simulink model "SWC_AFE_Control"  (R2022b)
settings: configuration reference "DC_DC_Charger_Configuration" (kept outside this file)
undefined symbols (not defined in the file or in its folder): DUTY_COUNT_LOWER_LMIT, DUTY_COUNT_UPPER_LMIT, Fault_Counts_perms, GRID_NORM_FREQ, GRID_VOLT_ADC_OFFSET, HALF_DUTY_PERIOD, INDUCTANCE, PI, PLL_FREQ_LOW_LIMIT, PLL_FREQ_UPP_LIMIT, PLL_PI_INTGRL_RESET, PLL_PI_KI, PLL_PI_KP, PLL_PI_LOWER_LIMIT, PLL_PI_UPPER_LIMIT, PLL_RATE, PLL_VD_ERROR_LIMIT, PLL_VD_ESTIMETED, PLL_VQ_ERROR_LIMIT, VDC_LOWER_LIM_SVPWM, VDC_UPPER_LIM_SVPWM
libraries: simulink x13, common_lib x8
(part 2 of 2)

== system SWC_AFE_Control/PWM_Loop/PLL/PLL_Lock_Detection_Block ==
  d_actual : Inport
  Vq_error : Inport  Port=2
  Abs : Abs  SaturateOnIntegerOverflow=off
  Abs1 : Abs  SaturateOnIntegerOverflow=off
  Add3 : Sum  Inputs=+-
  Constant1 : Constant  Value=PLL_VD_ESTIMETED  OutDataTypeStr=single  SampleTime=-1
  Constant12 : Constant  Value=PLL_VD_ERROR_LIMIT  OutDataTypeStr=single  SampleTime=-1
  Constant9 : Constant  Value=PLL_VQ_ERROR_LIMIT  OutDataTypeStr=single  SampleTime=-1
  Data Type Conversion : DataTypeConversion  OutDataTypeStr=single  SaturateOnIntegerOverflow=off  RndMeth=Floor
  Debounce1 : Subsystem  mask{Fault_Time_ms=40}
      mask DialogControl ParameterGroupVar Prompt: Fault Debounce time (msec)
  Logical Operator : Logic  AllPortsSameDT=off  OutDataTypeStr=boolean
  Relational Operator : RelationalOperator  Operator=<=  OutDataTypeStr=boolean  RndMeth=Simplest  InputSameDT=off
  Relational Operator2 : RelationalOperator  Operator=<=  OutDataTypeStr=boolean  RndMeth=Simplest  InputSameDT=off
  Switch2 : Switch  Threshold=0.5  SaturateOnIntegerOverflow=off  InputSameDT=off
  PLL_lock_out : Outport
  wires:
  Debounce1/1(Fault_Out) -> Switch2/1
  Switch2/1 -> PLL_lock_out/1
  Abs1/1 -> Relational Operator2/1
  Add3/1 -> Abs1/1
  Constant1/1 -> Add3/2
  d_actual/1 -> Add3/1
  Abs/1 -> Relational Operator/1
  Relational Operator/1 -> Logical Operator/2
  Relational Operator2/1 -> Logical Operator/1
  Constant12/1 -> Relational Operator2/2
  Constant9/1 -> Relational Operator/2
  Logical Operator/1 -> Data Type Conversion/1
  Vq_error/1 -> Abs/1
  Data Type Conversion/1 -> Debounce1/1(Fault_In), Switch2/2, Switch2/3

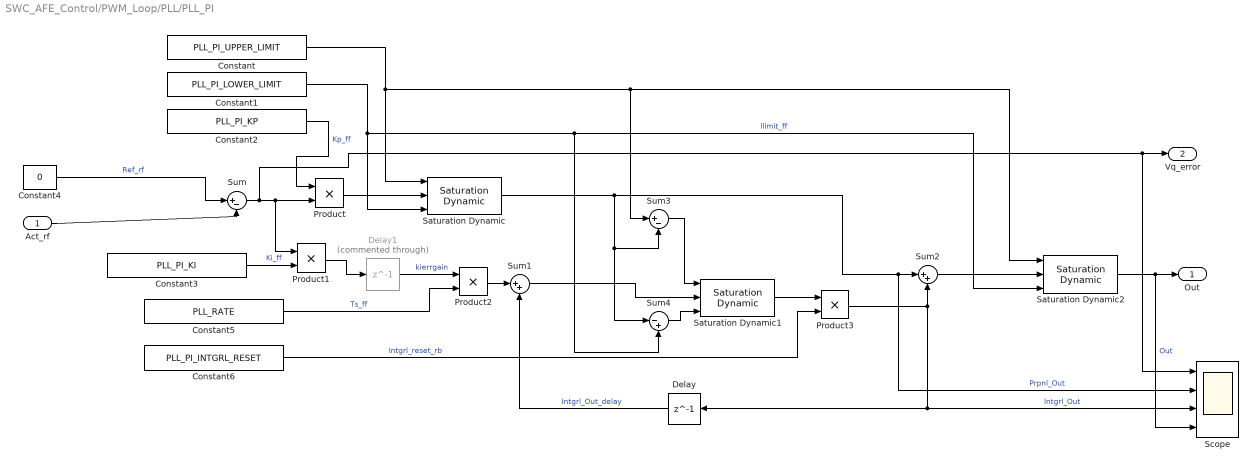
== system SWC_AFE_Control/PWM_Loop/PLL/PLL_PI ==
  Act_rf : Inport
  Constant : Constant  Value=PLL_PI_UPPER_LIMIT  SampleTime=-1
  Constant1 : Constant  Value=PLL_PI_LOWER_LIMIT  SampleTime=-1
  Constant2 : Constant  Value=PLL_PI_KP  SampleTime=-1
  Constant3 : Constant  Value=PLL_PI_KI  SampleTime=-1
  Constant4 : Constant  Value=0  SampleTime=-1
  Constant5 : Constant  Value=PLL_RATE  SampleTime=-1
  Constant6 : Constant  Value=PLL_PI_INTGRL_RESET  SampleTime=-1
  Delay : Delay  DelayLength=1
  Delay1 : Delay  Commented=through  DelayLength=1
  Product{,1..3} (4 alike) : Product
  Saturation Dynamic : simulink/Discontinuities/Saturation Dynamic  OutMin=[]  OutMax=[]  OutDataTypeStr=Inherit: Same as second input  OutDataType=fixdt(1, 16)  OutScaling=2^-10  DoSatur=off
  Saturation Dynamic1 : simulink/Discontinuities/Saturation Dynamic  OutMin=[]  OutMax=[]  OutDataTypeStr=Inherit: Same as second input  OutDataType=fixdt(1, 16)  OutScaling=2^-10  DoSatur=off
  Saturation Dynamic2 : simulink/Discontinuities/Saturation Dynamic  OutMin=[]  OutMax=[]  OutDataTypeStr=Inherit: Same as second input  OutDataType=fixdt(1, 16)  OutScaling=2^-10  DoSatur=off
  Scope : Scope  NumInputPorts=4
  Sum : Sum  Inputs=|+-
  Sum1 : Sum  Inputs=|++
  Sum2 : Sum  Inputs=|++
  Sum3 : Sum  Inputs=|+-
  Sum4 : Sum  Inputs=|-+
  Out : Outport
  Vq_error : Outport  Port=2
  wires:
  Sum/1 -> Scope/1, Vq_error/1, Product/2, Product1/1
  Constant5/1 -> Product2/2  "Ts_ff"
  Constant6/1 -> Product3/2  "Intgrl_reset_rb"
  Sum1/1 -> Saturation Dynamic1/2
  Product2/1 -> Sum1/1
  Product1/1 -> Delay1/1
  Saturation Dynamic2/1 -> Scope/4, Out/1  "Out"
  Delay1/1 -> Product2/1  "kierrgain"
  Saturation Dynamic1/1 -> Product3/1
  Sum3/1 -> Saturation Dynamic1/1
  Constant4/1 -> Sum/1  "Ref_rf"
  Sum4/1 -> Saturation Dynamic1/3
  Saturation Dynamic/1 -> Scope/2, Sum2/1, Sum3/2, Sum4/1  "Prpnl_Out"
  Delay/1 -> Sum1/2  "Intgrl_Out_delay"
  Sum2/1 -> Saturation Dynamic2/2
  Product/1 -> Saturation Dynamic/2
  Constant2/1 -> Product/1  "Kp_ff"
  Act_rf/1 -> Sum/2
  Product3/1 -> Scope/3, Delay/1, Sum2/2  "Intgrl_Out"
  Constant/1 -> Saturation Dynamic2/1, Sum3/1, Saturation Dynamic/1
  Constant3/1 -> Product1/2  "Ki_ff"
  Constant1/1 -> Sum4/2, Saturation Dynamic2/3, Saturation Dynamic/3  "llimit_ff"

== system SWC_AFE_Control/PWM_Loop/PLL/SOGI ==
  vg : Inport
  omega : Inport  Port=2
  Add : Sum  Inputs=+-  OutDataTypeStr=single
  Add1 : Sum
  Add2 : Sum  OutDataTypeStr=single
  Add3 : Sum  Inputs=-+  OutDataTypeStr=single
  Constant : Constant  Value=PLL_RATE  OutDataTypeStr=single  SampleTime=-1
  Delay{,1..3} (4 alike) : Delay  DelayLength=1
  Gain : Gain
  Product : Product
  Product1 : Product
  Product2 : Product
  vg_al : Outport
  vg_be : Outport  Port=2
  wires:
  omega/1 -> Product2/1  "omega"
  Product2/1 -> Product1/1, Product/2
  Constant/1 -> Product2/2
  Delay3/1 -> Add3/1
  Add3/1 -> Gain/1
  vg/1 -> Add3/2  "vg"
  Gain/1 -> Add/1
  Delay2/1 -> Add/2
  Delay1/1 -> Add2/1
  Product1/1 -> Add2/2
  Delay/1 -> Add1/2
  Product/1 -> Add1/1
  Add/1 -> Product/1
  Add1/1 -> vg_al/1, Delay3/1, Delay/1, Product1/2  "vg_al"
  Add2/1 -> vg_be/1, Delay1/1, Delay2/1  "vg_be"

== system SWC_AFE_Control/PWM_Loop/PLL/SOGI1 ==
  vg : Inport
  omega : Inport  Port=2
  Add : Sum  Inputs=+-  OutDataTypeStr=single
  Add1 : Sum
  Add2 : Sum  OutDataTypeStr=single
  Add3 : Sum  Inputs=-+  OutDataTypeStr=single
  Constant : Constant  Value=PLL_RATE  OutDataTypeStr=single  SampleTime=-1
  Delay{,1..3} (4 alike) : Delay  DelayLength=1
  Gain : Gain
  Product : Product
  Product1 : Product
  Product2 : Product
  vg_al : Outport
  vg_be : Outport  Port=2
  wires:
  Delay/1 -> Add1/2
  Delay3/1 -> Add3/1
  Gain/1 -> Add/1
  vg/1 -> Add3/2  "vg"
  Constant/1 -> Product2/2
  Add2/1 -> vg_be/1, Delay1/1, Delay2/1  "vg_be"
  Add3/1 -> Gain/1
  Product2/1 -> Product1/1, Product/2
  omega/1 -> Product2/1  "omega"
  Product1/1 -> Add2/2
  Product/1 -> Add1/1
  Delay2/1 -> Add/2
  Delay1/1 -> Add2/1
  Add/1 -> Product/1
  Add1/1 -> vg_al/1, Delay3/1, Delay/1, Product1/2  "vg_al"

== system SWC_AFE_Control/PWM_Loop/PLL/abctoalphabeta ==
  ph_a : Inport
  ph_b : Inport  Port=2
  ph_c : Inport  Port=3
  Gain1 : Gain  Gain=1/2
  Gain2 : Gain
  Gain3 : Gain  Gain=1/2
  Gain4 : Gain  Gain=sqrt(3)/2
  Sum : Sum  Inputs=|+--
  Sum5 : Sum  Inputs=|+-
  alpha : Outport
  beta : Outport  Port=2
  wires:
  Gain4/1 -> beta/1
  ph_a/1 -> Sum/1
  Gain3/1 -> Sum/3
  Gain2/1 -> alpha/1
  ph_c/1 -> Gain3/1, Sum5/2
  ph_b/1 -> Gain1/1, Sum5/1
  Sum5/1 -> Gain4/1
  Gain1/1 -> Sum/2
  Sum/1 -> Gain2/1

== system SWC_AFE_Control/PWM_Loop/PLL/alphabetatodq ==
  alpha : Inport
  beta : Inport  Port=2
  sinthetha : Inport  Port=3
  costhetha : Inport  Port=4
  Product{1..4} (4 alike) : Product
  Sum : Sum  Inputs=|++
  Sum5 : Sum  Inputs=|-+
  d : Outport
  q : Outport  Port=2
  wires:
  Product4/1 -> Sum5/2
  Product2/1 -> Sum5/1
  Product1/1 -> Sum/2
  Product3/1 -> Sum/1
  sinthetha/1 -> Product1/1, Product2/2
  beta/1 -> Product1/2, Product4/2
  costhetha/1 -> Product3/2, Product4/1
  alpha/1 -> Product3/1, Product2/1
  Sum5/1 -> q/1
  Sum/1 -> d/1

== system SWC_AFE_Control/PWM_Loop/PWM_DUTY/Subsystem ==
  In1 : Inport
  Add5 : Sum
  Constant7 : Constant  Value=HALF_DUTY_PERIOD
  Data Type Conversion : DataTypeConversion  OutDataTypeStr=single  SaturateOnIntegerOverflow=off  RndMeth=Floor
  Gain5 : Gain  Gain=HALF_DUTY_PERIOD
  Out1 : Outport
  wires:
  In1/1 -> Gain5/1
  Gain5/1 -> Add5/1
  Constant7/1 -> Add5/2
  Add5/1 -> Data Type Conversion/1
  Data Type Conversion/1 -> Out1/1

== system SWC_AFE_Control/PWM_Loop/PWM_DUTY/Subsystem1 ==
  In1 : Inport
  Add5 : Sum
  Constant7 : Constant  Value=HALF_DUTY_PERIOD
  Data Type Conversion : DataTypeConversion  OutDataTypeStr=single  SaturateOnIntegerOverflow=off  RndMeth=Floor
  Gain5 : Gain  Gain=HALF_DUTY_PERIOD
  Out1 : Outport
  wires:
  In1/1 -> Gain5/1
  Gain5/1 -> Add5/1
  Constant7/1 -> Add5/2
  Add5/1 -> Data Type Conversion/1
  Data Type Conversion/1 -> Out1/1

== system SWC_AFE_Control/PWM_Loop/PWM_DUTY/Subsystem2 ==
  In1 : Inport
  Add5 : Sum
  Constant7 : Constant  Value=HALF_DUTY_PERIOD
  Data Type Conversion : DataTypeConversion  OutDataTypeStr=single  SaturateOnIntegerOverflow=off  RndMeth=Floor
  Gain5 : Gain  Gain=HALF_DUTY_PERIOD
  Out1 : Outport
  wires:
  In1/1 -> Gain5/1
  Gain5/1 -> Add5/1
  Constant7/1 -> Add5/2
  Add5/1 -> Data Type Conversion/1
  Data Type Conversion/1 -> Out1/1

== system SWC_AFE_Control/Control_Loop/CONTROL/abctodq/abctoalphabeta ==
  ph_a : Inport
  ph_b : Inport  Port=2
  ph_c : Inport  Port=3
  Gain1 : Gain  Gain=1/2
  Gain2 : Gain  Gain=2/3
  Gain3 : Gain  Gain=1/2
  Gain4 : Gain  Gain=sqrt(3)/2*2/3
  Sum : Sum  Inputs=|+--
  Sum5 : Sum  Inputs=|+-
  alpha : Outport
  beta : Outport  Port=2
  wires:
  Sum/1 -> Gain2/1
  Gain1/1 -> Sum/2
  Sum5/1 -> Gain4/1
  ph_b/1 -> Sum5/1, Gain1/1
  ph_c/1 -> Sum5/2, Gain3/1
  Gain2/1 -> alpha/1
  Gain3/1 -> Sum/3
  ph_a/1 -> Sum/1
  Gain4/1 -> beta/1

== system SWC_AFE_Control/Control_Loop/CONTROL/abctodq/alphabetatodq ==
  alpha : Inport
  beta : Inport  Port=2
  sinthetha : Inport  Port=3
  costhetha : Inport  Port=4
  Product{1..4} (4 alike) : Product
  Sum : Sum  Inputs=|++
  Sum5 : Sum  Inputs=|-+
  d : Outport
  q : Outport  Port=2
  wires:
  Sum/1 -> d/1
  Sum5/1 -> q/1
  alpha/1 -> Product2/1, Product3/1
  costhetha/1 -> Product4/1, Product3/2
  beta/1 -> Product4/2, Product1/2
  sinthetha/1 -> Product2/2, Product1/1
  Product3/1 -> Sum/1
  Product1/1 -> Sum/2
  Product2/1 -> Sum5/1
  Product4/1 -> Sum5/2

== system SWC_AFE_Control/Control_Loop/CONTROL/dqtoabc/alphabetatoabc ==
  Input : Inport
  Input1 : Inport  Port=2
  Gain1 : Gain  Gain=sqrt(3)/2
  Gain3 : Gain  Gain=1/2
  Sum : Sum  Inputs=|+-  AccumDataTypeStr=single  OutDataTypeStr=single
  Sum5 : Sum  Inputs=|--  AccumDataTypeStr=single  OutDataTypeStr=single
  ph_a : Outport
  ph_b : Outport  Port=2
  ph_c : Outport  Port=3
  wires:
  Sum5/1 -> ph_c/1
  Input1/1 -> Gain1/1
  Input/1 -> Gain3/1, ph_a/1
  Sum/1 -> ph_b/1
  Gain1/1 -> Sum5/1, Sum/1
  Gain3/1 -> Sum/2, Sum5/2

== system SWC_AFE_Control/Control_Loop/CONTROL/dqtoabc/dqtoalphabeta ==
  Input2 : Inport
  Input3 : Inport  Port=2
  Input1 : Inport  Port=3
  Input : Inport  Port=4
  Product{1..4} (4 alike) : Product
  Sum : Sum  Inputs=|+-  AccumDataTypeStr=single  OutDataTypeStr=single
  Sum5 : Sum  Inputs=|++  AccumDataTypeStr=single  OutDataTypeStr=single
  alpha : Outport
  beta : Outport  Port=2
  wires:
  Sum/1 -> alpha/1
  Sum5/1 -> beta/1
  Input2/1 -> Product2/1, Product3/1
  Input/1 -> Product4/1, Product3/2
  Input3/1 -> Product4/2, Product1/2
  Input1/1 -> Product2/2, Product1/1
  Product3/1 -> Sum/1
  Product1/1 -> Sum/2
  Product2/1 -> Sum5/1
  Product4/1 -> Sum5/2

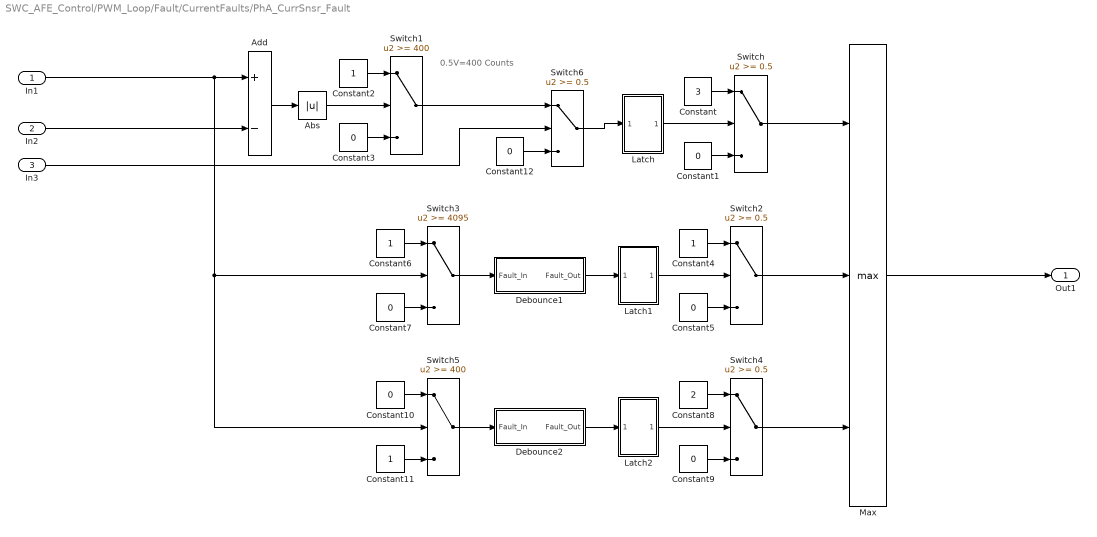
== system SWC_AFE_Control/PWM_Loop/Fault/CurrentFaults/PhA_CurrSnsr_Fault ==
  note: 0.5V=400 Counts
  In1 : Inport
  In2 : Inport  Port=2
  In3 : Inport  Port=3
  Abs : Abs  SaturateOnIntegerOverflow=off
  Add : Sum  Inputs=+-
  Constant : Constant  Value=3
  Constant{1,3,5,7,9..10,12} (7 alike) : Constant  Value=0
  Constant{2,4,6,11} (4 alike) : Constant
  Constant8 : Constant  Value=2
  Debounce1 : Subsystem  mask{Fault_Time_ms=4}
      mask DialogControl ParameterGroupVar Prompt: Fault Debounce time (msec)
  Debounce2 : Subsystem  mask{Fault_Time_ms=4}
      mask DialogControl ParameterGroupVar Prompt: Fault Debounce time (msec)
  Latch : Subsystem
  Latch1 : Subsystem
  Latch2 : Subsystem
  Max : MinMax  Function=max  Inputs=3
  Switch{,2,4,6} (4 alike) : Switch  Threshold=0.5  SaturateOnIntegerOverflow=off  InputSameDT=off
  Switch1 : Switch  Threshold=400  SaturateOnIntegerOverflow=off  InputSameDT=off
  Switch3 : Switch  Threshold=4095  SaturateOnIntegerOverflow=off  InputSameDT=off
  Switch5 : Switch  Threshold=400  SaturateOnIntegerOverflow=off  InputSameDT=off
  Out1 : Outport
  wires:
  Constant6/1 -> Switch3/1
  Switch1/1 -> Switch6/1
  Constant2/1 -> Switch1/1
  Switch/1 -> Max/1
  Constant7/1 -> Switch3/3
  Debounce1/1(Fault_Out) -> Latch1/1(In1)
  Switch3/1 -> Debounce1/1(Fault_In)
  Constant4/1 -> Switch2/1
  Latch1/1(Out1) -> Switch2/2
  Constant5/1 -> Switch2/3
  Switch6/1 -> Latch/1(In1)
  Add/1 -> Abs/1
  Constant/1 -> Switch/1
  Constant1/1 -> Switch/3
  Constant8/1 -> Switch4/1
  Constant11/1 -> Switch5/3
  Latch/1(Out1) -> Switch/2
  Constant9/1 -> Switch4/3
  Latch2/1(Out1) -> Switch4/2
  Debounce2/1(Fault_Out) -> Latch2/1(In1)
  In1/1 -> Switch5/2, Switch3/2, Add/1
  Switch4/1 -> Max/3
  Switch2/1 -> Max/2
  Constant3/1 -> Switch1/3
  Constant12/1 -> Switch6/3
  Switch5/1 -> Debounce2/1(Fault_In)
  Constant10/1 -> Switch5/1
  Abs/1 -> Switch1/2
  In2/1 -> Add/2
  Max/1 -> Out1/1
  In3/1 -> Switch6/2

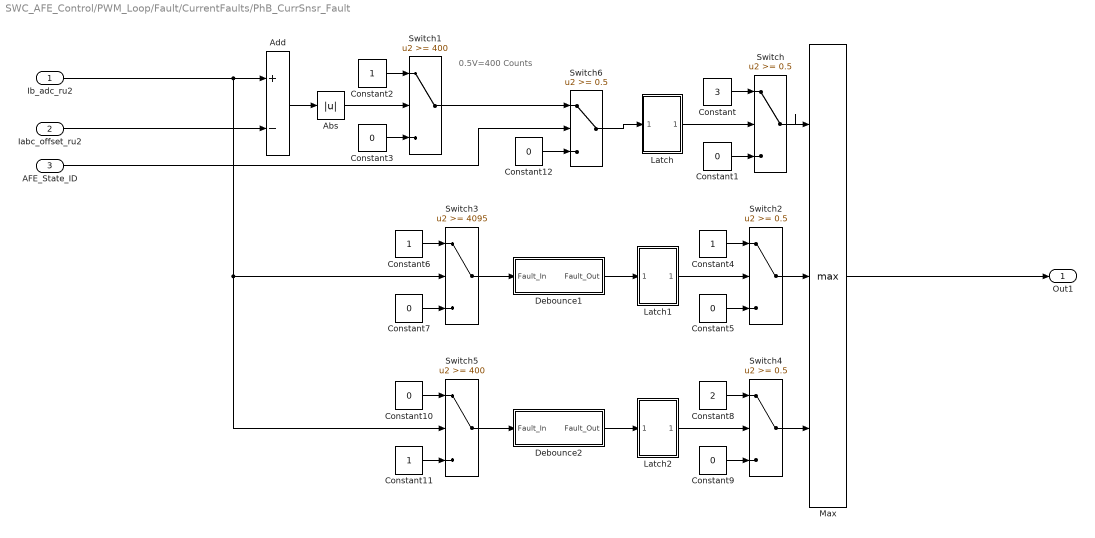
== system SWC_AFE_Control/PWM_Loop/Fault/CurrentFaults/PhB_CurrSnsr_Fault ==
  note: 0.5V=400 Counts
  Ib_adc_ru2 : Inport
  Iabc_offset_ru2 : Inport  Port=2
  AFE_State_ID : Inport  Port=3
  Abs : Abs  SaturateOnIntegerOverflow=off
  Add : Sum  Inputs=+-
  Constant : Constant  Value=3
  Constant{1,3,5,7,9..10,12} (7 alike) : Constant  Value=0
  Constant{2,4,6,11} (4 alike) : Constant
  Constant8 : Constant  Value=2
  Debounce1 : Subsystem  mask{Fault_Time_ms=4}
      mask DialogControl ParameterGroupVar Prompt: Fault Debounce time (msec)
  Debounce2 : Subsystem  mask{Fault_Time_ms=4}
      mask DialogControl ParameterGroupVar Prompt: Fault Debounce time (msec)
  Latch : Subsystem
  Latch1 : Subsystem
  Latch2 : Subsystem
  Max : MinMax  Function=max  Inputs=3
  Switch{,2,4,6} (4 alike) : Switch  Threshold=0.5  SaturateOnIntegerOverflow=off  InputSameDT=off
  Switch1 : Switch  Threshold=400  SaturateOnIntegerOverflow=off  InputSameDT=off
  Switch3 : Switch  Threshold=4095  SaturateOnIntegerOverflow=off  InputSameDT=off
  Switch5 : Switch  Threshold=400  SaturateOnIntegerOverflow=off  InputSameDT=off
  Out1 : Outport
  wires:
  Constant6/1 -> Switch3/1
  Switch1/1 -> Switch6/1
  Constant2/1 -> Switch1/1
  Switch/1 -> Max/1
  Constant7/1 -> Switch3/3
  Debounce1/1(Fault_Out) -> Latch1/1(In1)
  Switch3/1 -> Debounce1/1(Fault_In)
  Constant4/1 -> Switch2/1
  Latch1/1(Out1) -> Switch2/2
  Constant5/1 -> Switch2/3
  Switch6/1 -> Latch/1(In1)
  Add/1 -> Abs/1
  Constant/1 -> Switch/1
  Constant1/1 -> Switch/3
  Constant8/1 -> Switch4/1
  Constant11/1 -> Switch5/3
  Latch/1(Out1) -> Switch/2
  Constant9/1 -> Switch4/3
  Latch2/1(Out1) -> Switch4/2
  Debounce2/1(Fault_Out) -> Latch2/1(In1)
  Ib_adc_ru2/1 -> Switch5/2, Switch3/2, Add/1
  Switch4/1 -> Max/3
  Switch2/1 -> Max/2
  Constant3/1 -> Switch1/3
  Constant12/1 -> Switch6/3
  Switch5/1 -> Debounce2/1(Fault_In)
  Constant10/1 -> Switch5/1
  Abs/1 -> Switch1/2
  Iabc_offset_ru2/1 -> Add/2
  Max/1 -> Out1/1
  AFE_State_ID/1 -> Switch6/2

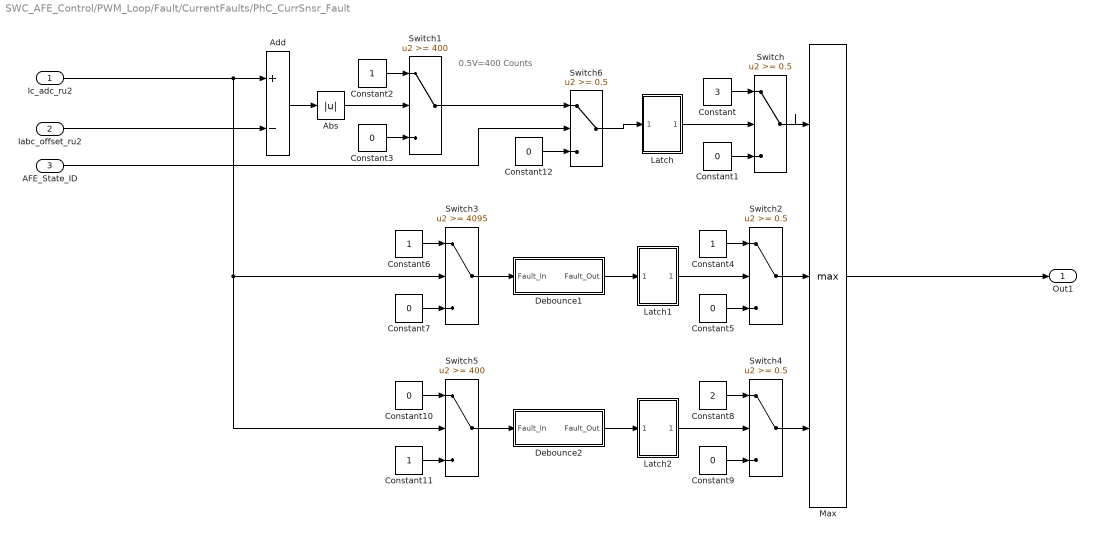
== system SWC_AFE_Control/PWM_Loop/Fault/CurrentFaults/PhC_CurrSnsr_Fault ==
  note: 0.5V=400 Counts
  Ic_adc_ru2 : Inport
  Iabc_offset_ru2 : Inport  Port=2
  AFE_State_ID : Inport  Port=3
  Abs : Abs  SaturateOnIntegerOverflow=off
  Add : Sum  Inputs=+-
  Constant : Constant  Value=3
  Constant{1,3,5,7,9..10,12} (7 alike) : Constant  Value=0
  Constant{2,4,6,11} (4 alike) : Constant
  Constant8 : Constant  Value=2
  Debounce1 : Subsystem  mask{Fault_Time_ms=4}
      mask DialogControl ParameterGroupVar Prompt: Fault Debounce time (msec)
  Debounce2 : Subsystem  mask{Fault_Time_ms=4}
      mask DialogControl ParameterGroupVar Prompt: Fault Debounce time (msec)
  Latch : Subsystem
  Latch1 : Subsystem
  Latch2 : Subsystem
  Max : MinMax  Function=max  Inputs=3
  Switch{,2,4,6} (4 alike) : Switch  Threshold=0.5  SaturateOnIntegerOverflow=off  InputSameDT=off
  Switch1 : Switch  Threshold=400  SaturateOnIntegerOverflow=off  InputSameDT=off
  Switch3 : Switch  Threshold=4095  SaturateOnIntegerOverflow=off  InputSameDT=off
  Switch5 : Switch  Threshold=400  SaturateOnIntegerOverflow=off  InputSameDT=off
  Out1 : Outport
  wires:
  Constant6/1 -> Switch3/1
  Switch1/1 -> Switch6/1
  Constant2/1 -> Switch1/1
  Switch/1 -> Max/1
  Constant7/1 -> Switch3/3
  Debounce1/1(Fault_Out) -> Latch1/1(In1)
  Switch3/1 -> Debounce1/1(Fault_In)
  Constant4/1 -> Switch2/1
  Latch1/1(Out1) -> Switch2/2
  Constant5/1 -> Switch2/3
  Switch6/1 -> Latch/1(In1)
  Add/1 -> Abs/1
  Constant/1 -> Switch/1
  Constant1/1 -> Switch/3
  Constant8/1 -> Switch4/1
  Constant11/1 -> Switch5/3
  Latch/1(Out1) -> Switch/2
  Constant9/1 -> Switch4/3
  Latch2/1(Out1) -> Switch4/2
  Debounce2/1(Fault_Out) -> Latch2/1(In1)
  Ic_adc_ru2/1 -> Switch5/2, Switch3/2, Add/1
  Switch4/1 -> Max/3
  Switch2/1 -> Max/2
  Constant3/1 -> Switch1/3
  Constant12/1 -> Switch6/3
  Switch5/1 -> Debounce2/1(Fault_In)
  Constant10/1 -> Switch5/1
  Abs/1 -> Switch1/2
  Iabc_offset_ru2/1 -> Add/2
  Max/1 -> Out1/1
  AFE_State_ID/1 -> Switch6/2

== system SWC_AFE_Control/PWM_Loop/PLL/Integrator/WrapRange ==
  Omega_1 : Inport
  range : Inport  Port=2
  Add : Sum  Inputs=-+
  Add1 : Sum  Inputs=+-
  Data Type Conversion : DataTypeConversion  OutDataTypeStr=int32  SaturateOnIntegerOverflow=off  RndMeth=Floor
  Divide : Product  Inputs=*/
  Divide1 : Product
  Gain : Gain  Gain=2
  Relational Operator : RelationalOperator  Operator=>  OutDataTypeStr=boolean  InputSameDT=off
  Switch1 : Switch  Threshold=0.5  SaturateOnIntegerOverflow=off  InputSameDT=off
  WRAP_ANGLE : Outport
  wires:
  Omega_1/1 -> Divide/1, Add1/1
  Gain/1 -> Divide1/2, Add/1, Divide/2  "2*range"
  range/1 -> Gain/1, Relational Operator/2
  Divide/1 -> Data Type Conversion/1
  Data Type Conversion/1 -> Divide1/1
  Divide1/1 -> Add1/2
  Add1/1 -> Relational Operator/1, Switch1/3, Add/2
  Relational Operator/1 -> Switch1/2
  Add/1 -> Switch1/1
  Switch1/1 -> WRAP_ANGLE/1

== system SWC_AFE_Control/PWM_Loop/PLL/PLL_Lock_Detection_Block/Debounce1 ==
  Fault_In : Inport
  Add : Sum
  Delay1 : Delay  DelayLength=1
  Product : Product
  Saturation : Saturate  UpperLimit=(Fault_Counts_perms * Fault_Time_ms)+1  LowerLimit=0
  Switch : Switch  Threshold=(Fault_Counts_perms * Fault_Time_ms)  SaturateOnIntegerOverflow=off  InputSameDT=off
  and : Logic  AllPortsSameDT=off  OutDataTypeStr=boolean
  one : Constant
  zero : Constant  Value=0
  Fault_Out : Outport  VectorParamsAs1DForOutWhenUnconnected=off
  wires:
  Switch/1 -> and/1
  Product/1 -> Delay1/1
  one/1 -> Switch/1
  Fault_In/1 -> Product/1, Add/1, and/2
  zero/1 -> Switch/3
  Saturation/1 -> Product/2, Switch/2
  Add/1 -> Saturation/1
  Delay1/1 -> Add/2
  and/1 -> Fault_Out/1

== system SWC_AFE_Control/PWM_Loop/Fault/CurrentFaults/PhA_CurrSnsr_Fault/Debounce1 ==
  Fault_In : Inport
  Add : Sum
  Delay1 : Delay  DelayLength=1
  Product : Product
  Saturation : Saturate  UpperLimit=(Fault_Counts_perms * Fault_Time_ms)+1  LowerLimit=0
  Switch : Switch  Threshold=(Fault_Counts_perms * Fault_Time_ms)  SaturateOnIntegerOverflow=off  InputSameDT=off
  and : Logic  AllPortsSameDT=off  OutDataTypeStr=boolean
  one : Constant
  zero : Constant  Value=0
  Fault_Out : Outport  VectorParamsAs1DForOutWhenUnconnected=off
  wires:
  and/1 -> Fault_Out/1
  Delay1/1 -> Add/2
  Add/1 -> Saturation/1
  Saturation/1 -> Switch/2, Product/2
  zero/1 -> Switch/3
  Fault_In/1 -> and/2, Add/1, Product/1
  one/1 -> Switch/1
  Product/1 -> Delay1/1
  Switch/1 -> and/1

== system SWC_AFE_Control/PWM_Loop/Fault/CurrentFaults/PhA_CurrSnsr_Fault/Debounce2 ==
  Fault_In : Inport
  Add : Sum
  Delay1 : Delay  DelayLength=1
  Product : Product
  Saturation : Saturate  UpperLimit=(Fault_Counts_perms * Fault_Time_ms)+1  LowerLimit=0
  Switch : Switch  Threshold=(Fault_Counts_perms * Fault_Time_ms)  SaturateOnIntegerOverflow=off  InputSameDT=off
  and : Logic  AllPortsSameDT=off  OutDataTypeStr=boolean
  one : Constant
  zero : Constant  Value=0
  Fault_Out : Outport  VectorParamsAs1DForOutWhenUnconnected=off
  wires:
  and/1 -> Fault_Out/1
  Delay1/1 -> Add/2
  Add/1 -> Saturation/1
  Saturation/1 -> Switch/2, Product/2
  zero/1 -> Switch/3
  Fault_In/1 -> and/2, Add/1, Product/1
  one/1 -> Switch/1
  Product/1 -> Delay1/1
  Switch/1 -> and/1

== system SWC_AFE_Control/PWM_Loop/Fault/CurrentFaults/PhA_CurrSnsr_Fault/Latch ==
  In1 : Inport
  Delay : Delay  DelayLength=1
  Flt_OR2 : Logic  Operator=OR  IconShape=distinctive  AllPortsSameDT=off  OutDataTypeStr=boolean
  Out1 : Outport
  wires:
  Delay/1 -> Flt_OR2/2
  Flt_OR2/1 -> Out1/1, Delay/1
  In1/1 -> Flt_OR2/1

== system SWC_AFE_Control/PWM_Loop/Fault/CurrentFaults/PhA_CurrSnsr_Fault/Latch1 ==
  In1 : Inport
  Delay : Delay  DelayLength=1
  Flt_OR2 : Logic  Operator=OR  IconShape=distinctive  AllPortsSameDT=off  OutDataTypeStr=boolean
  Out1 : Outport
  wires:
  Delay/1 -> Flt_OR2/2
  Flt_OR2/1 -> Out1/1, Delay/1
  In1/1 -> Flt_OR2/1

== system SWC_AFE_Control/PWM_Loop/Fault/CurrentFaults/PhA_CurrSnsr_Fault/Latch2 ==
  In1 : Inport
  Delay : Delay  DelayLength=1
  Flt_OR2 : Logic  Operator=OR  IconShape=distinctive  AllPortsSameDT=off  OutDataTypeStr=boolean
  Out1 : Outport
  wires:
  Delay/1 -> Flt_OR2/2
  Flt_OR2/1 -> Out1/1, Delay/1
  In1/1 -> Flt_OR2/1

== system SWC_AFE_Control/PWM_Loop/Fault/CurrentFaults/PhB_CurrSnsr_Fault/Debounce1 ==
  Fault_In : Inport
  Add : Sum
  Delay1 : Delay  DelayLength=1
  Product : Product
  Saturation : Saturate  UpperLimit=(Fault_Counts_perms * Fault_Time_ms)+1  LowerLimit=0
  Switch : Switch  Threshold=(Fault_Counts_perms * Fault_Time_ms)  SaturateOnIntegerOverflow=off  InputSameDT=off
  and : Logic  AllPortsSameDT=off  OutDataTypeStr=boolean
  one : Constant
  zero : Constant  Value=0
  Fault_Out : Outport  VectorParamsAs1DForOutWhenUnconnected=off
  wires:
  and/1 -> Fault_Out/1
  Delay1/1 -> Add/2
  Add/1 -> Saturation/1
  Saturation/1 -> Switch/2, Product/2
  zero/1 -> Switch/3
  Fault_In/1 -> and/2, Add/1, Product/1
  one/1 -> Switch/1
  Product/1 -> Delay1/1
  Switch/1 -> and/1

== system SWC_AFE_Control/PWM_Loop/Fault/CurrentFaults/PhB_CurrSnsr_Fault/Debounce2 ==
  Fault_In : Inport
  Add : Sum
  Delay1 : Delay  DelayLength=1
  Product : Product
  Saturation : Saturate  UpperLimit=(Fault_Counts_perms * Fault_Time_ms)+1  LowerLimit=0
  Switch : Switch  Threshold=(Fault_Counts_perms * Fault_Time_ms)  SaturateOnIntegerOverflow=off  InputSameDT=off
  and : Logic  AllPortsSameDT=off  OutDataTypeStr=boolean
  one : Constant
  zero : Constant  Value=0
  Fault_Out : Outport  VectorParamsAs1DForOutWhenUnconnected=off
  wires:
  and/1 -> Fault_Out/1
  Delay1/1 -> Add/2
  Add/1 -> Saturation/1
  Saturation/1 -> Switch/2, Product/2
  zero/1 -> Switch/3
  Fault_In/1 -> and/2, Add/1, Product/1
  one/1 -> Switch/1
  Product/1 -> Delay1/1
  Switch/1 -> and/1

== system SWC_AFE_Control/PWM_Loop/Fault/CurrentFaults/PhB_CurrSnsr_Fault/Latch ==
  In1 : Inport
  Delay : Delay  DelayLength=1
  Flt_OR2 : Logic  Operator=OR  IconShape=distinctive  AllPortsSameDT=off  OutDataTypeStr=boolean
  Out1 : Outport
  wires:
  Delay/1 -> Flt_OR2/2
  Flt_OR2/1 -> Out1/1, Delay/1
  In1/1 -> Flt_OR2/1

== system SWC_AFE_Control/PWM_Loop/Fault/CurrentFaults/PhB_CurrSnsr_Fault/Latch1 ==
  In1 : Inport
  Delay : Delay  DelayLength=1
  Flt_OR2 : Logic  Operator=OR  IconShape=distinctive  AllPortsSameDT=off  OutDataTypeStr=boolean
  Out1 : Outport
  wires:
  Delay/1 -> Flt_OR2/2
  Flt_OR2/1 -> Out1/1, Delay/1
  In1/1 -> Flt_OR2/1

== system SWC_AFE_Control/PWM_Loop/Fault/CurrentFaults/PhB_CurrSnsr_Fault/Latch2 ==
  In1 : Inport
  Delay : Delay  DelayLength=1
  Flt_OR2 : Logic  Operator=OR  IconShape=distinctive  AllPortsSameDT=off  OutDataTypeStr=boolean
  Out1 : Outport
  wires:
  Delay/1 -> Flt_OR2/2
  Flt_OR2/1 -> Out1/1, Delay/1
  In1/1 -> Flt_OR2/1

== system SWC_AFE_Control/PWM_Loop/Fault/CurrentFaults/PhC_CurrSnsr_Fault/Debounce1 ==
  Fault_In : Inport
  Add : Sum
  Delay1 : Delay  DelayLength=1
  Product : Product
  Saturation : Saturate  UpperLimit=(Fault_Counts_perms * Fault_Time_ms)+1  LowerLimit=0
  Switch : Switch  Threshold=(Fault_Counts_perms * Fault_Time_ms)  SaturateOnIntegerOverflow=off  InputSameDT=off
  and : Logic  AllPortsSameDT=off  OutDataTypeStr=boolean
  one : Constant
  zero : Constant  Value=0
  Fault_Out : Outport  VectorParamsAs1DForOutWhenUnconnected=off
  wires:
  and/1 -> Fault_Out/1
  Delay1/1 -> Add/2
  Add/1 -> Saturation/1
  Saturation/1 -> Switch/2, Product/2
  zero/1 -> Switch/3
  Fault_In/1 -> and/2, Add/1, Product/1
  one/1 -> Switch/1
  Product/1 -> Delay1/1
  Switch/1 -> and/1

== system SWC_AFE_Control/PWM_Loop/Fault/CurrentFaults/PhC_CurrSnsr_Fault/Debounce2 ==
  Fault_In : Inport
  Add : Sum
  Delay1 : Delay  DelayLength=1
  Product : Product
  Saturation : Saturate  UpperLimit=(Fault_Counts_perms * Fault_Time_ms)+1  LowerLimit=0
  Switch : Switch  Threshold=(Fault_Counts_perms * Fault_Time_ms)  SaturateOnIntegerOverflow=off  InputSameDT=off
  and : Logic  AllPortsSameDT=off  OutDataTypeStr=boolean
  one : Constant
  zero : Constant  Value=0
  Fault_Out : Outport  VectorParamsAs1DForOutWhenUnconnected=off
  wires:
  and/1 -> Fault_Out/1
  Delay1/1 -> Add/2
  Add/1 -> Saturation/1
  Saturation/1 -> Switch/2, Product/2
  zero/1 -> Switch/3
  Fault_In/1 -> and/2, Add/1, Product/1
  one/1 -> Switch/1
  Product/1 -> Delay1/1
  Switch/1 -> and/1

== system SWC_AFE_Control/PWM_Loop/Fault/CurrentFaults/PhC_CurrSnsr_Fault/Latch ==
  In1 : Inport
  Delay : Delay  DelayLength=1
  Flt_OR2 : Logic  Operator=OR  IconShape=distinctive  AllPortsSameDT=off  OutDataTypeStr=boolean
  Out1 : Outport
  wires:
  Delay/1 -> Flt_OR2/2
  Flt_OR2/1 -> Out1/1, Delay/1
  In1/1 -> Flt_OR2/1

== system SWC_AFE_Control/PWM_Loop/Fault/CurrentFaults/PhC_CurrSnsr_Fault/Latch1 ==
  In1 : Inport
  Delay : Delay  DelayLength=1
  Flt_OR2 : Logic  Operator=OR  IconShape=distinctive  AllPortsSameDT=off  OutDataTypeStr=boolean
  Out1 : Outport
  wires:
  Delay/1 -> Flt_OR2/2
  Flt_OR2/1 -> Out1/1, Delay/1
  In1/1 -> Flt_OR2/1

== system SWC_AFE_Control/PWM_Loop/Fault/CurrentFaults/PhC_CurrSnsr_Fault/Latch2 ==
  In1 : Inport
  Delay : Delay  DelayLength=1
  Flt_OR2 : Logic  Operator=OR  IconShape=distinctive  AllPortsSameDT=off  OutDataTypeStr=boolean
  Out1 : Outport
  wires:
  Delay/1 -> Flt_OR2/2
  Flt_OR2/1 -> Out1/1, Delay/1
  In1/1 -> Flt_OR2/1
